simulink model "lorentzsimu_control_obs"  (R2017b)
settings: Solver=ode4  StartTime=0.0  StopTime=15  FixedStep=1e-5  RelTol=1e-3
values from neighbouring files (symbols this model uses):
  A1 = Jnumerico1    [lorentzlqr.m]
  B1 = eye(3)    [lorentzlqr.m]
  beta = 2    [TEA_Ejercicios0_control_barco_sMatlab.m]    (also in lorentz.m = 2.66666666667; lorentzlqr.m = 2.66666666667)
  C1 = eye(3)    [lorentzlqr.m]
  D1 = zeros(3)    [lorentzlqr.m]
  init = Pnumerico(1,:)+1    [lorentzlqr.m]
  KClqr = lqr(A1,B1,Qc,Rc)    [lorentzlqr.m]
  Ko = KoT'    [lorentzlqr.m]
  Pnumerico = double(Psimbolico)    [lorentzlqr.m]
  rho = 28    [lorentz.m]    (also in lorentzlqr.m)
  sat = 5    [lorentzlqr.m]
  sigma = 10    [lorentz.m]    (also in lorentzlqr.m)
  tau_act = 0.01    [lorentzlqr.m]
settings Model: Creator=pablo  LastModifiedBy=pablo

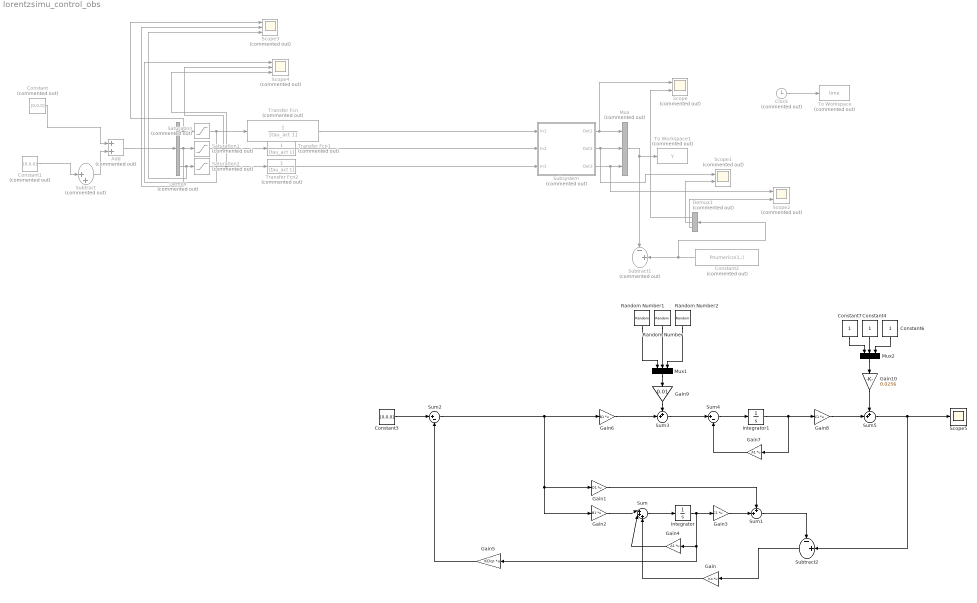
== system lorentzsimu_control_obs ==
  Add : Sum  Commented=on
  Clock : Clock  Commented=on
  Constant : Constant  Commented=on  Value=[0,0,0]
  Constant1 : Constant  Commented=on  Value=[0,0,0]
  Constant2 : Constant  Commented=on  Value=Pnumerico(1,:)
  Constant3 : Constant  Value=[0,0,0]
  Constant4 : Constant
  Constant6 : Constant
  Constant7 : Constant
  Demux : Demux  Commented=on  Outputs=3
  Demux1 : Demux  Commented=on  Outputs=3
  Gain : Gain  Gain=Ko  Multiplication=Matrix(K*u)
  Gain1 : Gain  Gain=D1  Multiplication=Matrix(K*u)
  Gain10 : Gain  Gain=0.0256
  Gain2 : Gain  Gain=B1  Multiplication=Matrix(K*u)
  Gain3 : Gain  Gain=C1  Multiplication=Matrix(K*u)
  Gain4 : Gain  Gain=A1  Multiplication=Matrix(K*u)
  Gain5 : Gain  Gain=KClqr  Multiplication=Matrix(K*u)
  Gain6 : Gain  Gain=B1  Multiplication=Matrix(K*u)
  Gain7 : Gain  Gain=A1  Multiplication=Matrix(K*u)
  Gain8 : Gain  Gain=C1  Multiplication=Matrix(K*u)
  Gain9 : Gain  Gain=0.01
  Integrator : Integrator
  Integrator1 : Integrator
  Mux : Mux  Commented=on  Inputs=3
  Mux1 : Mux  Inputs=3
  Mux2 : Mux  Inputs=3
  Random Number : RandomNumber  Variance=0.01*0.01  SampleTime=1e-5
  Random Number1 : RandomNumber  Variance=0.01*0.01  SampleTime=1e-5
  Random Number2 : RandomNumber  Variance=0.01*0.01  SampleTime=1e-5
  Saturation : Saturate  Commented=on  UpperLimit=sat  LowerLimit=-sat
  Saturation1 : Saturate  Commented=on  UpperLimit=sat  LowerLimit=-sat
  Saturation2 : Saturate  Commented=on  UpperLimit=sat  LowerLimit=-sat
  Scope : Scope  Commented=on  NumInputPorts=2
  Scope1 : Scope  Commented=on  NumInputPorts=2
  Scope2 : Scope  Commented=on  NumInputPorts=2
  Scope3 : Scope  Commented=on  NumInputPorts=3
  Scope4 : Scope  Commented=on  NumInputPorts=3
  Scope5 : Scope
  Subsystem : Subsystem  Commented=on
  Subtract : Sum  Commented=on  Inputs=|++
  Subtract1 : Sum  Commented=on  Inputs=-+|
  Subtract2 : Sum  Inputs=-+|
  Sum : Sum  Inputs=|+++
  Sum1 : Sum  Inputs=++|
  Sum2 : Sum  Inputs=|+-
  Sum3 : Sum  Inputs=++|
  Sum4 : Sum  Inputs=|+-
  Sum5 : Sum  Inputs=++|
  To Workspace : ToWorkspace  Commented=on  VariableName=time  SaveFormat=Timeseries  SampleTime=-1
  To Workspace1 : ToWorkspace  Commented=on  VariableName=Y  SaveFormat=Timeseries  SampleTime=-1
  Transfer Fcn : TransferFcn  Commented=on  Denominator=[tau_act 1]
  Transfer Fcn1 : TransferFcn  Commented=on  Denominator=[tau_act 1]
  Transfer Fcn2 : TransferFcn  Commented=on  Denominator=[tau_act 1]
  wires:
  Clock/1 -> To Workspace/1
  Demux/1 -> Saturation/1, Scope3/1
  Demux/2 -> Saturation1/1, Scope3/2
  Demux/3 -> Saturation2/1, Scope3/3
  Add/1 -> Demux/1
  Subsystem/1(Out1) -> Scope/1, Mux/1
  Subsystem/2(Out2) -> Scope1/1, Mux/2
  Subsystem/3(Out3) -> Scope2/1, Mux/3
  Mux/1 -> Subtract1/1, To Workspace1/1
  Subtract/1 -> Add/2
  Constant2/1 -> Subtract1/2, Demux1/1
  Constant/1 -> Add/1
  Constant1/1 -> Subtract/1
  Demux1/1 -> Scope/2
  Demux1/2 -> Scope1/2
  Demux1/3 -> Scope2/2
  Saturation/1 -> Transfer Fcn/1, Scope4/1
  Saturation1/1 -> Transfer Fcn1/1, Scope4/2
  Saturation2/1 -> Transfer Fcn2/1, Scope4/3
  Transfer Fcn/1 -> Subsystem/1(In1)
  Transfer Fcn1/1 -> Subsystem/2(In2)
  Transfer Fcn2/1 -> Subsystem/3(In3)
  Gain3/1 -> Sum1/2
  Sum/1 -> Integrator/1
  Gain4/1 -> Sum/2
  Integrator/1 -> Gain5/1, Gain4/1, Gain3/1
  Gain/1 -> Sum/3
  Sum1/1 -> Subtract2/1
  Gain1/1 -> Sum1/1
  Gain2/1 -> Sum/1
  Subtract2/1 -> Gain/1
  Constant3/1 -> Sum2/1
  Sum2/1 -> Gain2/1, Gain1/1, Gain6/1
  Gain6/1 -> Sum3/2
  Sum3/1 -> Sum4/1
  Sum4/1 -> Integrator1/1
  Gain7/1 -> Sum4/2
  Integrator1/1 -> Gain7/1, Gain8/1
  Gain8/1 -> Sum5/2
  Gain10/1 -> Sum5/1
  Sum5/1 -> Subtract2/2, Scope5/1
  Random Number/1 -> Mux1/2
  Mux1/1 -> Gain9/1
  Random Number1/1 -> Mux1/1
  Random Number2/1 -> Mux1/3
  Gain9/1 -> Sum3/1
  Constant4/1 -> Mux2/2
  Mux2/1 -> Gain10/1
  Constant6/1 -> Mux2/3
  Constant7/1 -> Mux2/1
  Gain5/1 -> Sum2/2

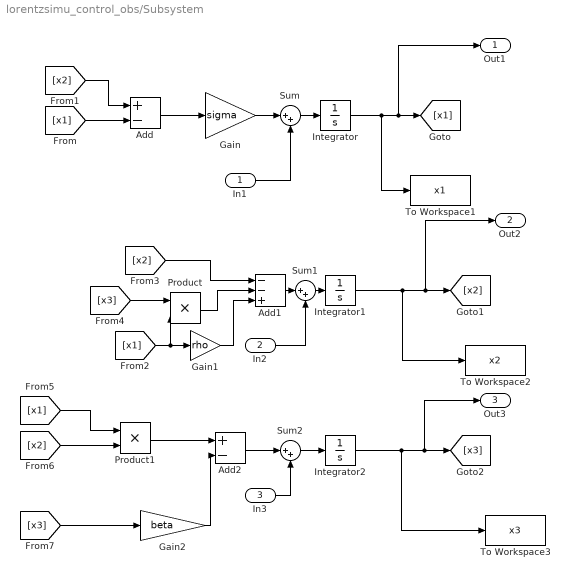
== system lorentzsimu_control_obs/Subsystem ==
  In1 : Inport
  In2 : Inport  Port=2
  In3 : Inport  Port=3
  Add : Sum  Inputs=+-
  Add1 : Sum  Inputs=--+
  Add2 : Sum  Inputs=+-
  Gain : Gain  Gain=sigma
  Gain1 : Gain  Gain=rho
  Gain2 : Gain  Gain=beta
  Integrator : Integrator  InitialCondition=init(1)
  Integrator1 : Integrator  InitialCondition=init(2)
  Integrator2 : Integrator  InitialCondition=init(3)
  Product : Product
  Product1 : Product
  Sum : Sum  Inputs=|++
  Sum1 : Sum  Inputs=|++
  Sum2 : Sum  Inputs=|++
  To Workspace1 : ToWorkspace  VariableName=x1  SampleTime=-1
  To Workspace2 : ToWorkspace  VariableName=x2  SampleTime=-1
  To Workspace3 : ToWorkspace  VariableName=x3  SampleTime=-1
  Out1 : Outport
  Out2 : Outport  Port=2
  Out3 : Outport  Port=3
  wires:
  [x1] -> Product/2, Gain1/1
  Integrator/1 -> To Workspace1/1, Out1/1, [x1]
  [x2] -> Add/1
  [x1] -> Add/2
  Add/1 -> Gain/1
  Gain1/1 -> Add1/3
  [x2] -> Add1/1
  Product/1 -> Add1/2
  [x3] -> Product/1
  Integrator1/1 -> To Workspace2/1, Out2/1, [x2]
  Product1/1 -> Add2/1
  [x1] -> Product1/1
  [x2] -> Product1/2
  [x3] -> Gain2/1
  Gain2/1 -> Add2/2
  Integrator2/1 -> To Workspace3/1, Out3/1, [x3]
  Gain/1 -> Sum/1
  Sum/1 -> Integrator/1
  In1/1 -> Sum/2
  Add1/1 -> Sum1/1
  Sum1/1 -> Integrator1/1
  In2/1 -> Sum1/2
  In3/1 -> Sum2/2
  Add2/1 -> Sum2/1
  Sum2/1 -> Integrator2/1
